simulink library "libAircraftWingFusalageSpecs"  (R2020b)
settings: Solver=VariableStepAuto  StartTime=0.0  StopTime=10.0  RelTol=1e-3
undefined symbols (not defined in the file): data
settings Model: Creator=caatay  LastModifiedBy=caatay

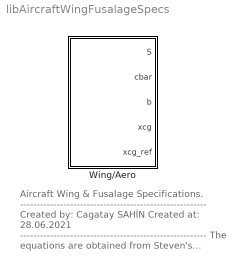
== system libAircraftWingFusalageSpecs ==
  note: Aircraft Wing & Fusalage
      | Specifications.
      | --------------------------------------------------------
      | Created by: Cagatay SAHİN
      | Created at: 28.06.2021
      | --------------------------------------------------------
      | The equations are obtained from
      | Steven's textbook.
      | The reference book can be found in
      | "references folder".
      | --------------------------------------------------------
      | for question:
      | cagataysahin44@gmail.com
  Wing/Aero : Subsystem  mask(Aircraft Specifications - Wing and Fusalage Specifications){S=data.acSpec.wing.S, cbar=data.acSpec.wing.cbar, b=data.acSpec.wing.b, xcg=data.acSpec.fusalage.x_cg, xcg_ref=data.acSpec.fusalage.x_cg_ref}
      mask prompts: S "Wing Area"; cbar "Mean Aerodynamic Chord"; b "Wing Span"; xcg "Center of Gravity"; xcg_ref "Nominal Center of Gravity"
      mask help: Aircraft wing and fusalage specifications to use in equation of motions.
      mask Help:
      | This block is used for getting aircraft's wing and fusalage specifications in Imperic system.
      | --------------------------------------------------------------------------------------------------------------------------------------------------
      | Output of the function:
      | 	S: Wing Reference Area (ft^2)
      | 	cbar: Mean Aerodynamic Chord (ft)
      |                   b: Wing Span (ft)
      |                   x_cg: Fusalage center of gravitiy position on x-axis (ft)
      | 	x_cg_ref: Fusalage nominal center of gravity position on x-axis (ft)
      | --------------------------------------------------------------------------------------------------------------------------------------------------
      | All equations can be found in Steven's text book. Reference can be found in "literature" subfolder.
      | for question: "cagataysahin44@gmail.com"
      mask Display:
      | port_label('output',1,'S','texmode','on');
      | port_label('output',2,'cbar','texmode','on');
      | port_label('output',3,'b','texmode','on');
      | port_label('output',4,'x_{cg}','texmode','on');
      | port_label('output',5,'x_{cg_{ref}}','texmode','on');

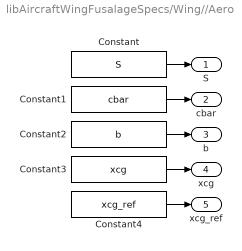
== system libAircraftWingFusalageSpecs/Wing//Aero ==
  Constant : Constant  Value=S
  Constant1 : Constant  Value=cbar
  Constant2 : Constant  Value=b
  Constant3 : Constant  Value=xcg
  Constant4 : Constant  Value=xcg_ref
  S : Outport  VectorParamsAs1DForOutWhenUnconnected=off
  cbar : Outport  Port=2  VectorParamsAs1DForOutWhenUnconnected=off
  b : Outport  Port=3  VectorParamsAs1DForOutWhenUnconnected=off
  xcg : Outport  Port=4  VectorParamsAs1DForOutWhenUnconnected=off
  xcg_ref : Outport  Port=5  VectorParamsAs1DForOutWhenUnconnected=off
  wires:
  Constant3/1 -> xcg/1
  Constant4/1 -> xcg_ref/1
  Constant2/1 -> b/1
  Constant1/1 -> cbar/1
  Constant/1 -> S/1
